simulink model "problem_4"  (R2020b)
settings: Solver=VariableStepAuto  StartTime=0.0  StopTime=10.0  RelTol=1e-3
settings Model: Creator=hp  LastModifiedBy=hp

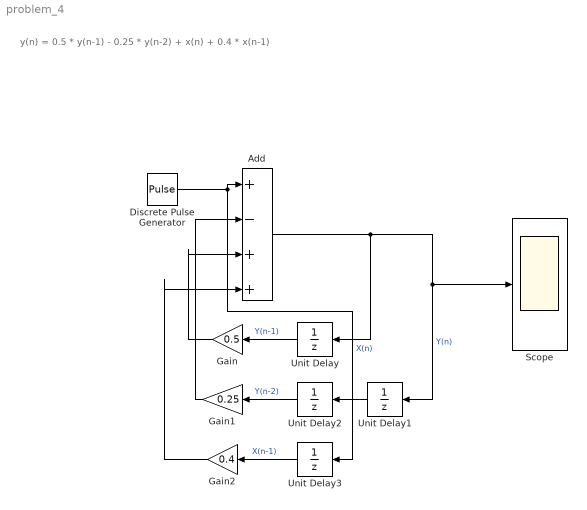
== system problem_4 ==
  note: y(n) = 0.5 * y(n-1) - 0.25 * y(n-2) + x(n) + 0.4 * x(n-1)
  Add : Sum  Inputs=+-++
  Discrete Pulse Generator : DiscretePulseGenerator  Period=10  PulseWidth=5
  Gain : Gain  Gain=0.5
  Gain1 : Gain  Gain=0.25
  Gain2 : Gain  Gain=0.4
  Scope : Scope
  Unit Delay{,1..3} (4 alike) : UnitDelay  SampleTime=-1  HasFrameUpgradeWarning=on
  wires:
  Discrete Pulse Generator/1 -> Unit Delay3/1, Add/1  "X(n)"
  Gain/1 -> Add/3
  Gain1/1 -> Add/2
  Gain2/1 -> Add/4
  Add/1 -> Scope/1, Unit Delay1/1, Unit Delay/1  "Y(n)"
  Unit Delay/1 -> Gain/1  "Y(n-1)"
  Unit Delay1/1 -> Unit Delay2/1
  Unit Delay2/1 -> Gain1/1  "Y(n-2)"
  Unit Delay3/1 -> Gain2/1  "X(n-1)"
